simulink model "test"  (R2023b)
settings: Solver=FixedStepAuto  StartTime=0.0  StopTime=10.0  FixedStep=5e-7  RelTol=1e-3
libraries: spsSawtoothGeneratorLib x1
settings Model: Creator=LZQ  LastModifiedBy=LZQ
settings SolverCC: AllowMultiTaskInputOutput=on  ConcurrentTasks=on

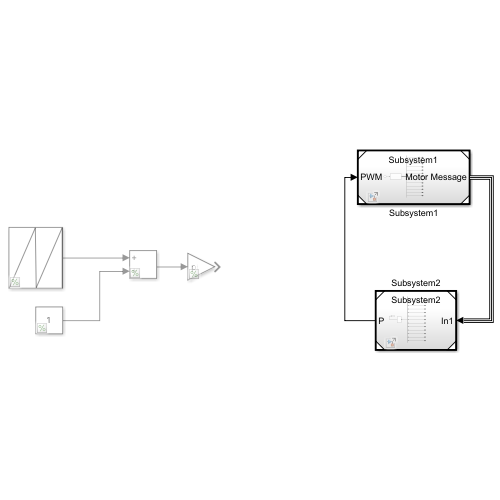
[thumbnail: Simulink's stored preview of the top-level diagram]
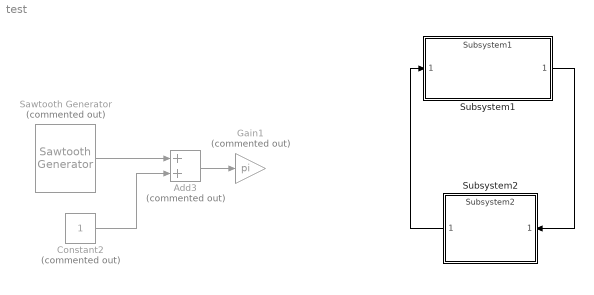
== system test ==
  Add3 : Sum  Commented=on
  Constant2 : Constant  Commented=on
  Gain1 : Gain  Commented=on  Gain=pi
  Sawtooth Generator : spsSawtoothGeneratorLib/Sawtooth Generator  Commented=on  Freq=1  Phase=360  Ts=0
  Subsystem1 : ModelReference  ModelNameDialog=Subsystem1  SimulationMode=Normal  ModelReferenceVersion=1.3
  Subsystem2 : ModelReference  ModelNameDialog=Subsystem2  SimulationMode=Normal  ModelReferenceVersion=1.6
  wires:
  Constant2/1 -> Add3/2
  Add3/1 -> Gain1/1
  Sawtooth Generator/1 -> Add3/1
  Subsystem1/1 -> Subsystem2/1
  Subsystem2/1 -> Subsystem1/1
